simulink model "FILE"  (R2024a)
settings: Solver=VariableStepAuto  StartTime=0.0  StopTime=15  FixedStep=0.1  RelTol=1e-3
values from neighbouring files (symbols this model uses):
  A = [-(F/V)-K_0*exp(-E_over_R / T)  ,- K_0 * C_A * exp(-E_over_R / T)/T^2*(-E_over_R) ... (first row only)    [LYAP.m]    (also in MAIN.m; modello.m = [-(F/V)-K_0*exp(-E_over_R / T)  ,-(-E_over_R)*K_0 * C_A * ex)
  B = [0; 3.377]    [MAIN.m]    (also in modello.m)
  bin_u = [-50 -40 -30 -20 -10 0 10 20 30 40 50]    [bin_u.mat]
  bin_x1 = [0 0.142857142857 0.285714285714 0.5 338.6 0.6 0.857142857143 1]    [bin_x1.mat]
  bin_x2 = [300 310 320 330 340 350 360 370 380 390 400]    [bin_x2.mat]
  Qtable = [nan 0.778416671354 -259.126360869 -700.115558265 nan -896.463806415 nan nan 0.47295513559 0.108400525713 -655.424557632 -739.208275844 ... (968 elements, 8x11x11)]    [Q4.mat]    (also in Q5.mat = [nan 0.692639901098 0.879438132945 -140.341088423 nan -330.7)
  Tabella = []    [MAIN.m]
undefined symbols (not defined in the file or in its folder): sigbuilder_block
libraries: slpidlib x2
settings Model: Creator=Strix  LastModifiedBy=Strix
settings DebuggingCC: OperatingPointInterfaceChecksumMismatchMsg=none

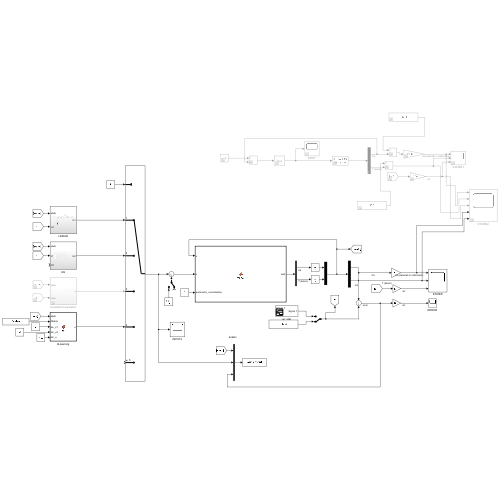
[thumbnail: Simulink's stored preview of the top-level diagram]
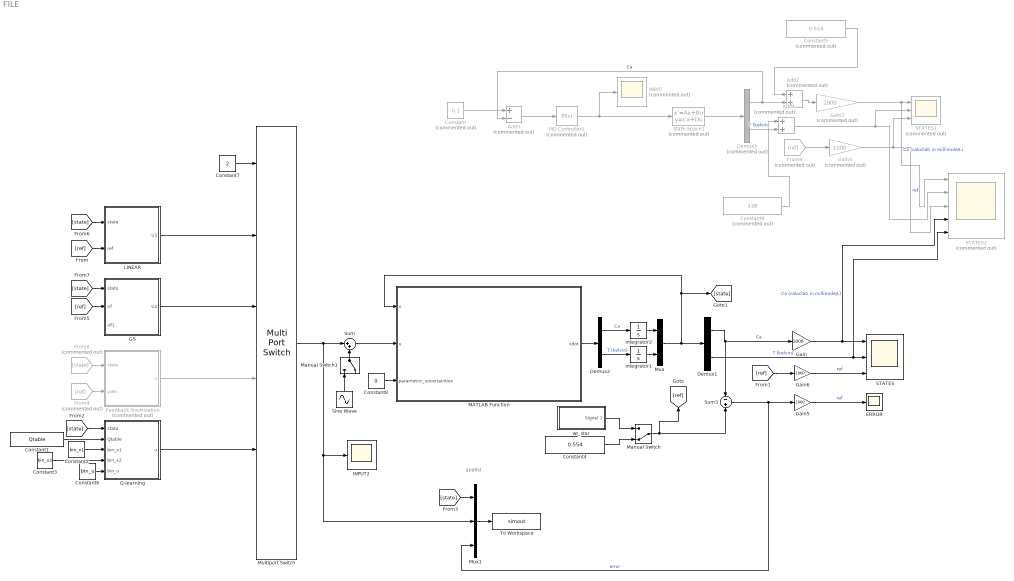
== system FILE ==
  note: analisi
  Add2 : Sum  Commented=on
  Add3 : Sum  Commented=on  Inputs=+-
  Add4 : Sum  Commented=on
  Constant : Constant  Commented=on  Value=0.1
  Constant1 : Constant  Value=Qtable
  Constant2 : Constant  Value=bin_x1
  Constant3 : Constant  Value=bin_x2
  Constant4 : Constant  Value=0.554
  Constant5 : Constant  Commented=on  Value=0.554
  Constant6 : Constant  Value=bin_u
  Constant7 : Constant  Value=2
  Constant8 : Constant  Value=0
  Constant9 : Constant  Commented=on  Value=338
  Demux1 : Demux  Outputs=2
  Demux2 : Demux  Outputs=2
  Demux3 : Demux  Commented=on  Outputs=2
  ERROR : Scope
  Feedback linearization : Subsystem  Commented=on
  From4 : From  Commented=on  GotoTag=ref
  From8 : From  Commented=on  GotoTag=state
  From9 : From  Commented=on  GotoTag=ref
  GS : Subsystem
  Gain : Gain  Gain=1000
  Gain2 : Gain  Commented=on  Gain=1000
  Gain3 : Gain  Commented=on  Gain=1000
  Gain5 : Gain  Gain=1000
  Gain6 : Gain  Gain=1000
  INPUT : Scope  Commented=on
  INPUT2 : Scope
  Integrator1 : Integrator  InitialCondition=350
  Integrator2 : Integrator  InitialCondition=1
  LINEAR : Subsystem
  MATLAB Function : MATLAB Function  TreatAsAtomicUnit=on  SystemSampleTime=0.0001
  Manual Switch : ManualSwitch  CurrentSetting=0
  Manual Switch1 : ManualSwitch  CurrentSetting=0
  Multiport Switch : MultiPortSwitch  Inputs=5  SaturateOnIntegerOverflow=off  InputSameDT=off
  Mux : Mux  Inputs=2
  Mux1 : Mux  Inputs=3
  PID Controller2 : slpidlib/PID Controller  Commented=on  Controller=PI  Form=Parallel  TimeDomain=Continuous-time  UseExternalTs=off  SampleTime=-1  IntegratorMethod=Forward Euler  FilterMethod=Forward Euler  ControllerParametersSource=internal  P=-9  I=1  UseKiTs=off  D=0  UseExternalDerivativeSource=off  N=100  UseFilter=on  TunerSelectOption=Transfer Function Based (PID Tuner App)  InitialConditionSource=internal  InitialConditionForIntegrator=0  InitialConditionForFilter=0  DifferentiatorICPrevScaledInput=0  ExternalReset=none  TrackingMode=off  Kt=1  LimitOutput=off  SatLimitsSource=internal  UpperSaturationLimit=inf  LowerSaturationLimit=-inf  LinearizeAsGain=on  AntiWindupMode=none  Kb=1  LimitIntegrator=off  UpperIntegratorSaturationLimit=inf  LowerIntegratorSaturationLimit=-inf  POutMin=[]  POutMax=[]  IOutMin=[]  IOutMax=[]  DOutMin=[]  DOutMax=[]  NOutMin=[]  NOutMax=[]  SumOutMin=[]  SumOutMax=[]  SaturationOutMin=[]  SaturationOutMax=[]  PParamMin=[]  PParamMax=[]  IParamMin=[]  IParamMax=[]  DParamMin=[]  DParamMax=[]  NParamMin=[]  NParamMax=[]  KbParamMin=[]  KbParamMax=[]  KtParamMin=[]  KtParamMax=[]  KbOutMin=[]  KbOutMax=[]  KtOutMin=[]  KtOutMax=[]  IntegratorOutMin=[]  IntegratorOutMax=[]  FilterOutMin=[]  FilterOutMax=[]  SumI1OutMin=[]  SumI1OutMax=[]  SumI2OutMin=[]  SumI2OutMax=[]  SumI3OutMin=[]  SumI3OutMax=[]  SumI4OutMin=[]  SumI4OutMax=[]  SumDOutMin=[]  SumDOutMax=[]  DifferentiatorOutMin=[]  DifferentiatorOutMax=[]  FilterDiffOutCoefMin=[]  FilterDiffOutCoefMax=[]  ReciprocalOutMin=[]  ReciprocalOutMax=[]  SumDenOutMin=[]  SumDenOutMax=[]  SumNumOutMin=[]  SumNumOutMax=[]  DivideOutMin=[]  DivideOutMax=[]  UdiffTsProdOutMin=[]  UdiffTsProdOutMax=[]  NTsProdOutMin=[]  NTsProdOutMax=[]  UintegralTsProdOutMin=[]  UintegralTsProdOutMax=[]  UngainTsProdOutMin=[]  UngainTsProdOutMax=[]  ClampingZeroOutDataTypeStr=Inherit: Inherit via back propagation  ClampingZeroOutMin=[]  ClampingZeroOutMax=[]  FilterDenConstantOutDataTypeStr=Inherit: Inherit via back propagation  FilterDenConstantOutMin=[]  FilterDenConstantOutMax=[]  PCopyOutDataTypeStr=Inherit: Inherit via back propagation  PCopyOutMin=[]  PCopyOutMax=[]  NCopyOutDataTypeStr=Inherit: Inherit via back propagation  NCopyOutMin=[]  NCopyOutMax=[]  IntegratorContinuousStateAttributes=''  IntegratorStateMustResolveToSignalObject=off  IntegratorRTWStateStorageClass=Auto  FilterContinuousStateAttributes=''  FilterStateMustResolveToSignalObject=off  FilterRTWStateStorageClass=Auto  ParallelPVariant=InternalParameters  IdealPVariant=Disabled  IVariant=InternalParameters  DVariant=Disabled  IntegratorVariant=Continuous  SatVariant=Disabled  AWVariant=Passthrough  PCopyVariant=Disabled  TRVariant=Disabled  FdbkBlocksVariant=Forward  IdealPFdbkVariant=Disabled  SatFdbkVariant=Disabled  DerivativeFilterVariant=Disabled  NVariant=Disabled  NCopyVariant=Disabled_SignalSpec  FilterICVariant=Disabled  IntegratorICVariant=InternalICs  ExternalResetVariant=Disabled  TRSumVariant=Passthrough  SumFdbkVariant=Disabled  SumVariant=Sum_PI  TsampFilterVariant=InternalTs  TsampNgainVariant=Passthrough  TsampIntegralVariant=Disabled_SignalSpec  ExternalSaturationOutDataTypeStr=Inherit: Same as second input  DerivativeSourceVariant=Disabled
  Q-learning : MATLAB Function  TreatAsAtomicUnit=on  SystemSampleTime=0.0001
  STATES : Scope  NumInputPorts=3
  STATES1 : Scope  Commented=on  NumInputPorts=3
  STATES2 : Scope  Commented=on  NumInputPorts=5
  Sine Wave : Sin  Amplitude=5  Frequency=10  SampleTime=0
  State-Space1 : StateSpace  Commented=on  A=A  B=B  C=eye(2)  D=[0 0 ]'  InitialCondition=[0.1;0]
  Sum : Sum  Inputs=|++
  Sum3 : Sum  Inputs=-+
  To Workspace : ToWorkspace  VariableName=simout  SampleTime=-1
  wr_star : Subsystem  Tag=STV Subsys  LoadFcn=sigbuilder_block('load');  StartFcn=sigbuilder_block('start');  StopFcn=sigbuilder_block('stop');  ClipboardFcn=sigbuilder_block('clipboard');  mask(Sigbuilder block){tuvar=[0:10]}
      mask help: Simulink:masks:SigbuilderBlock_MD
      mask init:
      | if ~strcmp(get_param(bdroot(gcbh),'SimulationStatus'),'stopped') tuvar = sigbuilder_block('maskInit'); end
      settings: CopyFcn=sigbuilder_block('copy');  DeleteFcn=sigbuilder_block('delete');  ModelCloseFcn=sigbuilder_block('modelClose');  PreSaveFcn=sigbuilder_block('preSave');  PauseFcn=sigbuilder_block('pause');  ContinueFcn=sigbuilder_block('continue');  NameChangeFcn=sigbuilder_block('namechange');  OpenFcn=sigbuilder_block('open',[340 222 1141 580.5 ]);  CloseFcn=sigbuilder_block('close');
      mask Display: plot(0, 0, 100, 100,[2, 2, 32, 32, 2], [68, 8, 8, 68, 68],[32, 2], [38, 38], [32, 19, 2],[53, 60, 44], [32, 17, 17, 2],[16, 16, 31, 31]);txt = getActiveGroup(gcbh);text(2, 100, txt,'verticalAlignment', 'top');
  wires:
  Demux1/2 -> STATES2/5, STATES/2  "T (kelvin)"
  Demux1/1 -> Sum3/1, Gain/1  "Ca"
  Sum3/1 -> Mux1/3, Gain5/1  "error"
  Gain/1 -> STATES2/4, STATES/1  "Ca (caloclati in millimole/L)"
  [ref] -> Gain6/1
  Gain6/1 -> STATES/3  "ref"
  From4/1 -> Feedback linearization/2(ydes)
  State-Space1/1 -> Demux3/1
  Demux2/1 -> Integrator2/1  "Ca"
  Integrator2/1 -> Mux/1
  Demux2/2 -> Integrator1/1  "T (kelvin)"
  MATLAB Function/1(xdot) -> Demux2/1
  Mux/1 -> Demux1/1, MATLAB Function/1(x), [state]
  Multiport Switch/1 -> Sum/1, Mux1/2, INPUT2/1
  GS/1(U2) -> Multiport Switch/3
  Feedback linearization/1(u) -> Multiport Switch/4
  [ref] -> GS/2(rif)
  [state] -> GS/1(stato)
  From8/1 -> Feedback linearization/1(stato)
  Manual Switch/1 -> [ref], Sum3/2
  Gain5/1 -> ERROR/1  "ref"
  wr_star/1(Signal 1) -> Manual Switch/1
  Constant4/1 -> Manual Switch/2
  Integrator1/1 -> Mux/2
  Constant1/1 -> Q-learning/2(Qtable)
  [state] -> Q-learning/1(stato)
  Constant2/1 -> Q-learning/3(bin_x1)
  Constant3/1 -> Q-learning/4(bin_x2)
  Constant6/1 -> Q-learning/5(bin_u)
  Q-learning/1(u) -> Multiport Switch/5
  Constant7/1 -> Multiport Switch/1
  [state] -> Mux1/1
  Mux1/1 -> To Workspace/1
  Gain2/1 -> STATES2/1, STATES1/1  "Ca (caloclati in millimole/L)"
  Gain3/1 -> STATES2/3, STATES1/3  "ref"
  Sum/1 -> MATLAB Function/2(u)
  Add2/1 -> Gain2/1
  Demux3/1 -> Add3/2, Add2/2  "Ca"
  Constant5/1 -> Add2/1
  Constant/1 -> Add3/1
  From9/1 -> Gain3/1
  PID Controller2/1 -> INPUT/1, State-Space1/1
  Add3/1 -> PID Controller2/1
  Demux3/2 -> Add4/2  "T (kelvin)"
  Constant9/1 -> Add4/1
  Add4/1 -> STATES2/2, STATES1/2
  [ref] -> LINEAR/2(ref)
  [state] -> LINEAR/1(state)
  LINEAR/1(U1) -> Multiport Switch/2
  Manual Switch1/1 -> Sum/2
  Sine Wave/1 -> Manual Switch1/1
  Constant8/1 -> MATLAB Function/3(parametric_uncertainties)

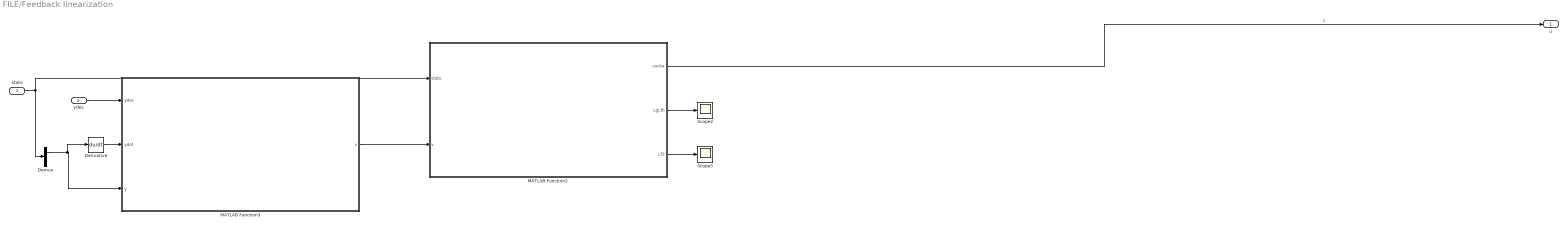
== system FILE/Feedback linearization ==
  stato : Inport
  ydes : Inport  Port=2
  Demux : Demux  Outputs=2
  Derivative : Derivative
  MATLAB Function2 : MATLAB Function  TreatAsAtomicUnit=on
  MATLAB Function3 : MATLAB Function  TreatAsAtomicUnit=on
  Scope2 : Scope
  Scope5 : Scope
  u : Outport
  wires:
  MATLAB Function2/3(Lf2) -> Scope5/1
  stato/1 -> MATLAB Function2/1(stato), Demux/1
  MATLAB Function2/2(LgLfh) -> Scope2/1
  Demux/1 -> Derivative/1, MATLAB Function3/3(y)
  MATLAB Function3/1(v) -> MATLAB Function2/2(v)
  Derivative/1 -> MATLAB Function3/2(ydot)
  ydes/1 -> MATLAB Function3/1(ydes)
  MATLAB Function2/1(uscita) -> u/1  "u"

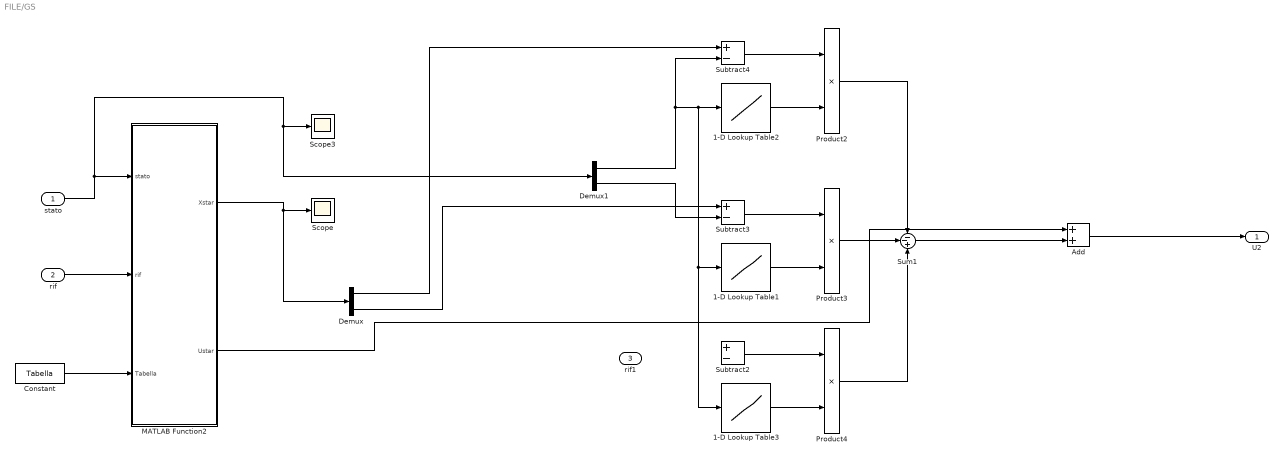
== system FILE/GS ==
  stato : Inport
  rif : Inport  Port=2
  rif1 : Inport  Port=3
  1-D Lookup Table1 : Lookup_n-D  NumberOfTableDimensions=1  BreakpointsForDimension1=flip(Tabella(:,2))  Table=flip((Tabella(:,5)))  InternalRulePriority=Speed  RndMeth=Simplest
  1-D Lookup Table2 : Lookup_n-D  NumberOfTableDimensions=1  BreakpointsForDimension1=flip(Tabella(:,2))  Table=flip((Tabella(:,4)))  InternalRulePriority=Speed  RndMeth=Simplest
  1-D Lookup Table3 : Lookup_n-D  NumberOfTableDimensions=1  BreakpointsForDimension1=flip(Tabella(:,2))  Table=flip((Tabella(:,6)))  InternalRulePriority=Speed  RndMeth=Simplest
  Add : Sum
  Constant : Constant  Value=Tabella
  Demux : Demux  Outputs=2
  Demux1 : Demux  Outputs=2
  MATLAB Function2 : MATLAB Function  TreatAsAtomicUnit=on
  Product2 : Product
  Product3 : Product
  Product4 : Product
  Scope : Scope
  Scope3 : Scope
  Subtract2 : Sum  Inputs=+-
  Subtract3 : Sum  Inputs=+-
  Subtract4 : Sum  Inputs=+-
  Sum1 : Sum  Inputs=--+
  U2 : Outport
  wires:
  Add/1 -> U2/1
  stato/1 -> Scope3/1, Demux1/1, MATLAB Function2/1(stato)
  1-D Lookup Table2/1 -> Product2/2
  1-D Lookup Table1/1 -> Product3/2
  1-D Lookup Table3/1 -> Product4/2
  MATLAB Function2/1(Xstar) -> Scope/1, Demux/1
  MATLAB Function2/2(Ustar) -> Add/1
  Product2/1 -> Sum1/1
  Product3/1 -> Sum1/2
  Product4/1 -> Sum1/3
  Sum1/1 -> Add/2
  Subtract2/1 -> Product4/1
  Demux/1 -> Subtract4/1
  Subtract3/1 -> Product3/1
  Subtract4/1 -> Product2/1
  Demux/2 -> Subtract3/1
  Demux1/1 -> 1-D Lookup Table1/1, 1-D Lookup Table3/1, 1-D Lookup Table2/1, Subtract4/2
  Demux1/2 -> Subtract3/2
  rif/1 -> MATLAB Function2/2(rif)
  Constant/1 -> MATLAB Function2/3(Tabella)

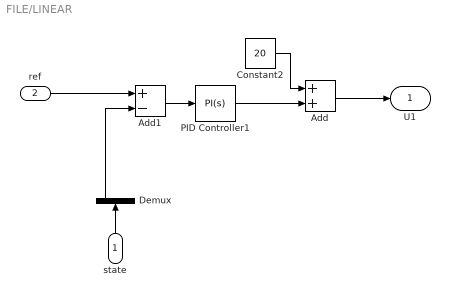
== system FILE/LINEAR ==
  state : Inport
  ref : Inport  Port=2
  Add : Sum
  Add1 : Sum  Inputs=+-
  Constant2 : Constant  Value=20
  Demux : Demux  Outputs=2
  PID Controller1 : slpidlib/PID Controller  Controller=PI  Form=Parallel  TimeDomain=Continuous-time  UseExternalTs=off  SampleTime=-1  IntegratorMethod=Forward Euler  FilterMethod=Forward Euler  ControllerParametersSource=internal  P=-9  I=-4  UseKiTs=off  D=0  UseExternalDerivativeSource=off  N=100  UseFilter=on  TunerSelectOption=Transfer Function Based (PID Tuner App)  InitialConditionSource=internal  InitialConditionForIntegrator=0  InitialConditionForFilter=0  DifferentiatorICPrevScaledInput=0  ExternalReset=none  TrackingMode=off  Kt=1  LimitOutput=off  SatLimitsSource=internal  UpperSaturationLimit=inf  LowerSaturationLimit=-inf  LinearizeAsGain=on  AntiWindupMode=none  Kb=1  LimitIntegrator=off  UpperIntegratorSaturationLimit=inf  LowerIntegratorSaturationLimit=-inf  POutMin=[]  POutMax=[]  IOutMin=[]  IOutMax=[]  DOutMin=[]  DOutMax=[]  NOutMin=[]  NOutMax=[]  SumOutMin=[]  SumOutMax=[]  SaturationOutMin=[]  SaturationOutMax=[]  PParamMin=[]  PParamMax=[]  IParamMin=[]  IParamMax=[]  DParamMin=[]  DParamMax=[]  NParamMin=[]  NParamMax=[]  KbParamMin=[]  KbParamMax=[]  KtParamMin=[]  KtParamMax=[]  KbOutMin=[]  KbOutMax=[]  KtOutMin=[]  KtOutMax=[]  IntegratorOutMin=[]  IntegratorOutMax=[]  FilterOutMin=[]  FilterOutMax=[]  SumI1OutMin=[]  SumI1OutMax=[]  SumI2OutMin=[]  SumI2OutMax=[]  SumI3OutMin=[]  SumI3OutMax=[]  SumI4OutMin=[]  SumI4OutMax=[]  SumDOutMin=[]  SumDOutMax=[]  DifferentiatorOutMin=[]  DifferentiatorOutMax=[]  FilterDiffOutCoefMin=[]  FilterDiffOutCoefMax=[]  ReciprocalOutMin=[]  ReciprocalOutMax=[]  SumDenOutMin=[]  SumDenOutMax=[]  SumNumOutMin=[]  SumNumOutMax=[]  DivideOutMin=[]  DivideOutMax=[]  UdiffTsProdOutMin=[]  UdiffTsProdOutMax=[]  NTsProdOutMin=[]  NTsProdOutMax=[]  UintegralTsProdOutMin=[]  UintegralTsProdOutMax=[]  UngainTsProdOutMin=[]  UngainTsProdOutMax=[]  ClampingZeroOutDataTypeStr=Inherit: Inherit via back propagation  ClampingZeroOutMin=[]  ClampingZeroOutMax=[]  FilterDenConstantOutDataTypeStr=Inherit: Inherit via back propagation  FilterDenConstantOutMin=[]  FilterDenConstantOutMax=[]  PCopyOutDataTypeStr=Inherit: Inherit via back propagation  PCopyOutMin=[]  PCopyOutMax=[]  NCopyOutDataTypeStr=Inherit: Inherit via back propagation  NCopyOutMin=[]  NCopyOutMax=[]  IntegratorContinuousStateAttributes=''  IntegratorStateMustResolveToSignalObject=off  IntegratorRTWStateStorageClass=Auto  FilterContinuousStateAttributes=''  FilterStateMustResolveToSignalObject=off  FilterRTWStateStorageClass=Auto  ParallelPVariant=InternalParameters  IdealPVariant=Disabled  IVariant=InternalParameters  DVariant=Disabled  IntegratorVariant=Continuous  SatVariant=Disabled  AWVariant=Passthrough  PCopyVariant=Disabled  TRVariant=Disabled  FdbkBlocksVariant=Forward  IdealPFdbkVariant=Disabled  SatFdbkVariant=Disabled  DerivativeFilterVariant=Disabled  NVariant=Disabled  NCopyVariant=Disabled_SignalSpec  FilterICVariant=Disabled  IntegratorICVariant=InternalICs  ExternalResetVariant=Disabled  TRSumVariant=Passthrough  SumFdbkVariant=Disabled  SumVariant=Sum_PI  TsampFilterVariant=InternalTs  TsampNgainVariant=Passthrough  TsampIntegralVariant=Disabled_SignalSpec  ExternalSaturationOutDataTypeStr=Inherit: Same as second input  DerivativeSourceVariant=Disabled
  U1 : Outport
  wires:
  PID Controller1/1 -> Add/2
  Add/1 -> U1/1
  ref/1 -> Add1/1
  Demux/1 -> Add1/2
  state/1 -> Demux/1
  Add1/1 -> PID Controller1/1
  Constant2/1 -> Add/1

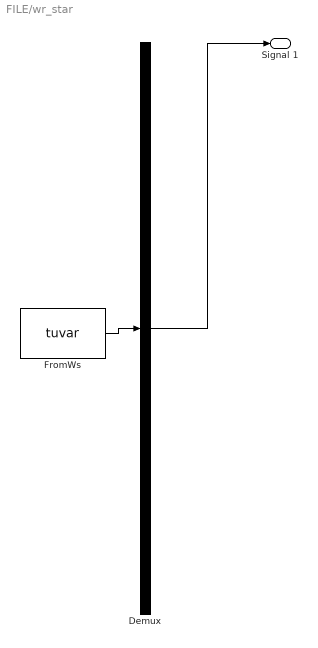
== system FILE/wr_star ==
  Demux : Demux  Tag=STV Demux  Outputs=1
      settings: DisplayOption=none
  FromWs : FromWorkspace  Tag=STV FromWs  VariableName=tuvar
      SigBuilderData=|
      | common.afterFinalStr = 'Extrapolate'
      | common.sampleTime = 0
      | dataSet.timeRange = [0 20]
      | dataSet.name = 'Group 1'
      | sbobj.Groups.Name = 'Group 1'
      | sbobj.Groups.Signals.Name = 'Signal 1'
      | sbobj.Groups.Signals.XData = [0 2.999 3 5.999 6 11 11 20]
      | sbobj.Groups.Signals.YData = [0.7151 0.7151 0.554 0.554 0.15 0.15 0.715 0.7151]
      | sbobj.Groups.TimeRange = [0 20]
  Signal 1 : Outport  Tag=STV Outport  VectorParamsAs1DForOutWhenUnconnected=off
  wires:
  Demux/1 -> Signal 1/1
  FromWs/1 -> Demux/1

== matlab function FILE/MATLAB Function ==
  data: x input; u input; xdot output; parametric_uncertainties input
function xdot  = model(x, u,parametric_uncertainties)
  
C_A = x(1); % Concentration of component A in outlet stream (mole/l)
T = x(2); % Temperature of the reactants in the reactor (K)
u; % Temperature of the coolant water in the jacket (K)

% Reactor Parameters
V = 50; % Reactor volume (l)
F= 50; % Inlet volumetric flow rate to the reactor (l/min)
C_A0 = 1; % Feed concentration of component A (mole/l)
K_0 = 7.8e10; % Pre-exponential factor (l/min)
E_over_R = 8567; % Activation energy in the Arrhenius equation (Cal/mole)
R = 1.987; % Universal gas constant (Cal/mole.K), assuming typical value
rho = 900; % Density of the inlet and outlet stream (g/l)
C_p = 0.329; % Heat capacity of inlet and outlet stream (Cal/g.K)
T_in = 350; % Inlet stream temperature (K)
H_r = -5e4; % Heat of reaction (Cal/mole)
UA = 5e4; % Heat transfer term (Cal/min.K)
rho_c = 1000; % Density of the coolant water in the jacket (g/l)
T_amb=293; %Temperatura ambiente (K)

if(parametric_uncertainties==1)
rho=rho*1.4;
end

    % Calcolo delle derivate
    x1dot = (F/V) *(C_A0 - C_A) - K_0 * C_A * exp(-E_over_R / T); %Cadot
    x2dot = (F/V) * (T_in - T)- (K_0 * C_A *  H_r)* exp(-E_over_R / T) / (rho * C_p)  - (UA / (rho * V * C_p)) * ( T- (T_amb+u));


 xdot=[x1dot, x2dot]';

 %X1=1-x(1)-7.8*10^10*x(1)*exp(-8567/x(2));

 %X2 = 1339.761 + 1.317e13 * C_A * exp(-8567 / T) - 4.377 * T + 3.377 * u;
%XX=[X1, X2]';

end

== matlab function FILE/Feedback linearization/MATLAB Function2 ==
  data: stato input; uscita output; v input; LgLfh output; Lf2 output
function [uscita,LgLfh ,Lf2]= fcn(stato,v)

x=stato(1);
y=stato(2);

V = 50; % Reactor volume (l)
F= 50; % Inlet volumetric flow rate to the reactor (l/min)
C_A0 = 1; % Feed concentration of component A (mole/l)
K_0 = 7.8e10; % Pre-exponential factor (l/min)
E_over_R = 8567; % Activation energy in the Arrhenius equation (Cal/mole)
R = 1.987; % Universal gas constant (Cal/mole.K), assuming typical value
rho = 900; % Density of the inlet and outlet stream (g/l)
C_p = 0.329; % Heat capacity of inlet and outlet stream (Cal/g.K)
T_in = 350; % Inlet stream temperature (K)
H_r = -5e4; % Heat of reaction (Cal/mole)
UA = 5e4; % Heat transfer term (Cal/min.K)
rho_c = 1000; % Density of the coolant water in the jacket (g/l)
T_amb=293; %Temperatura ambiente (K)

k=K_0;
u=0;
c=C_A0;
t=T_in;
a=1;
m=K_0*H_r/(rho*C_p);
g=T_amb;
s=UA/(rho*C_p*V);
R=E_over_R;

% Definisce x come variabile simbolica

LgLfh=(exp(-(2*R)/y)* k* R* (2* x* (m *x *(R - y) + k *y^2) + exp(R/y) *(-g *s* x* (R - 2* y) - s *x *(R* (u - y) + y* (-2* u + y)) + a *(R *x *(-t + y) + y *(2 *t* x - c*y + x* y)))))/y^4;

F1= a*(c-x)-k*x*exp(-R/y);
F2= a*(t-y)-m*x*exp(-R/y)-s*(y-g-u);


Lfdx=a^2 + (exp(-(2*R)/y) *k*(2* m *R* x + k* y^2))/y^2 + (exp(-R/y) *k* (-g* R* s + R* s* (-u + y) + a *(-R *t + R *y + 2* y^2)))/y^2;

Lfdy= (exp(-(2* R)/y) *k* R *(2* x *(m *x* (R - y) + k* y^2) + exp(R/y) *(-g *s* x* (R - 2* y) - s *x*(R* (u - y) + y* (-2* u + y)) + a *(R* x* (-t + y) + y* (2 *t* x - c *y *+ x* y)))))/y^4;





Lf2=[Lfdx Lfdy]*[F1 F2]';


uscita=(-Lf2+v)/LgLfh;

== matlab function FILE/Feedback linearization/MATLAB Function3 ==
  data: ydes input; v output; ydot input; y input
function v = fcn(ydes,ydot,y)
kd=1;
kp=1000;
v=kd*(0-ydot)+kp*(ydes-y);

== matlab function FILE/GS/MATLAB Function2 ==
  data: stato input; rif input; Xstar output; Ustar output; Tabella input
function [Xstar,Ustar]  = gains_computation(stato,rif,Tabella)


[~, idxgoal] = min(abs(Tabella(:,2) - rif));
[~, idx1] = min(abs(Tabella(:,2) - stato(1)));
if(idx1==idxgoal)
idx1=idx1;
elseif(idx1<idxgoal)
idx1=idx1+1;
else
idx1=idx1-1;
end

u=Tabella(idx1,1);
C_A =   Tabella(idx1,2)    ;        % Concentration of component A in outlet stream (mole/l)
T =    Tabella(idx1,3)   ;         % Temperature of the reactants in the reactor (K)
Xstar = [Tabella(idx1,2),Tabella(idx1,3)];
Ustar = Tabella(idx1,1);




end

== matlab function FILE/Q-learning ==
  data: stato input; Qtable input; u output; bin_x1 input; bin_x2 input; bin_u input
function u  = fcn(stato,Qtable,bin_x1,bin_x2,bin_u)
  

    [~, yDiscrx1] = min(abs(stato(1) - bin_x1));
    [~, yDiscrx2] = min(abs(stato(2) - bin_x2));
    [~, act_idx] = max(Qtable(yDiscrx1,yDiscrx2,:)); % Pick always greedy action
    u = bin_u(act_idx);

end
